simulink model "mechanical_system"  (R2015a)
settings: Solver=ode23t  StartTime=0.0  StopTime=10.0  RelTol=1e-3  AbsTol=1e-3
libraries: fl_lib x10, nesl_utility x4
settings Model: Creator=sseshadr  LastModifiedBy=sseshadr
settings SimscapeCC: SimscapeLogType=all  SimscapeLogDataHistory=10000

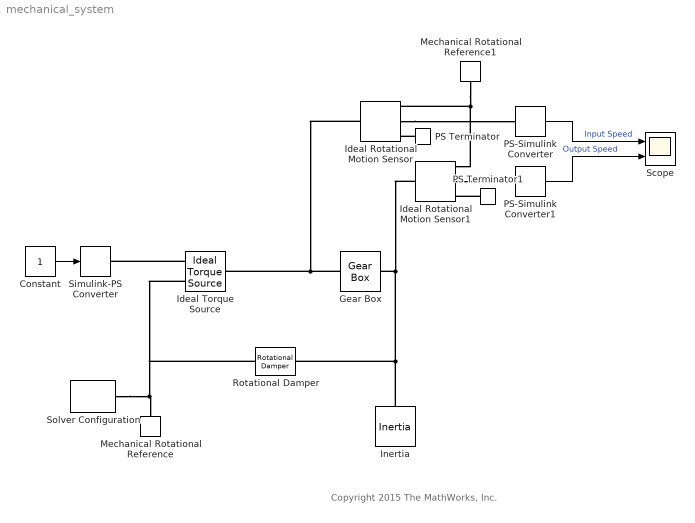
== system mechanical_system ==
  note: Copyright 2015 The MathWorks, Inc.
  Constant : Constant
  Gear Box : fl_lib/Mechanical/Mechanisms/Gear Box  ratio=2  t_in_specify=off  t_in_priority=High  t_in=0 N*m  t_out_specify=off  t_out_priority=High  t_out=0 N*m
  Ideal Rotational Motion Sensor : fl_lib/Mechanical/Mechanical Sensors/Ideal Rotational Motion Sensor  offset=0 rad
  Ideal Rotational Motion Sensor1 : fl_lib/Mechanical/Mechanical Sensors/Ideal Rotational Motion Sensor  offset=0 rad
  Ideal Torque Source : fl_lib/Mechanical/Mechanical Sources/Ideal Torque Source
  Inertia : fl_lib/Mechanical/Rotational Elements/Inertia  inertia=0.01 kg*m^2  w_specify=on  w_priority=High  w=10 rad/s  t_specify=off  t_priority=High  t=0 N*m
  Mechanical Rotational Reference : fl_lib/Mechanical/Rotational Elements/Mechanical Rotational Reference
  Mechanical Rotational Reference1 : fl_lib/Mechanical/Rotational Elements/Mechanical Rotational Reference
  PS Terminator : fl_lib/Physical Signals/Sinks/PS Terminator
  PS Terminator1 : fl_lib/Physical Signals/Sinks/PS Terminator
  PS-Simulink Converter : nesl_utility/PS-Simulink Converter  PhysicalDomain=network_engine_domain  SubClassName=ps_output  LeftPortType=input  RightPortType=output  PseudoPeriodic=off  Frequencies=[]  Unit=1  AffineConversion=off
  PS-Simulink Converter1 : nesl_utility/PS-Simulink Converter  PhysicalDomain=network_engine_domain  SubClassName=ps_output  LeftPortType=input  RightPortType=output  PseudoPeriodic=off  Frequencies=[]  Unit=1  AffineConversion=off
  Rotational Damper : fl_lib/Mechanical/Rotational Elements/Rotational Damper  D=0.001 N*m/(rad/s)  w_specify=off  w_priority=High  w=0 rad/s  t_specify=off  t_priority=High  t=0 N*m
  Scope : Scope  NumInputPorts=2
      settings: YMin=-5~-5  YMax=5~5
  Simulink-PS Converter : nesl_utility/Simulink-PS Converter  PhysicalDomain=network_engine_domain  SubClassName=ps_input  LeftPortType=input  RightPortType=output  PseudoPeriodic=off  Frequencies=[]  NoiseDistribution=none  NoiseParameters=[]  Unit=1  AffineConversion=off  InputFiltering=off  SimscapeFilterOrder=1  InputFilterTimeConstant=0.001  UdotUserProvided=1
  Solver Configuration : nesl_utility/Solver Configuration  PhysicalDomain=network_engine_domain  SubClassName=solver  LeftPortType=input  RightPortType=generic  Accelerate=off  Tones=[]  Harmonics=[]  SimulateNoise=off  Profile=off  UseLocalSampling=off  EnableSwitchedLinearOptims=on  FrequencyDomain=off  UseCCode=off  RelTol=0.001  AbsTol=1e-06  MinStep=1e-09  ToWorkspace=off  RevertToSquareIcSolve=off  NumHomotopyIterations=100  DoDC=off  ResidualTolerance=1e-09  UseLocalSolver=off  LocalSolverChoice=NE_BACKWARD_EULER_ADVANCER  LocalSolverSampleTime=0.001  DoFixedCost=off  MaxNonlinIter=3  MaxModeIter=2  LinearAlgebra=Sparse  DelaysMemoryBudget=1024  AutomaticFiltering=on  FilteringTimeConstant=0.001
  wires:
  PS-Simulink Converter/1 -> Scope/1  "Input Speed"
  Constant/1 -> Simulink-PS Converter/1
  PS-Simulink Converter1/1 -> Scope/2  "Output Speed"
  connections:
  Ideal Torque Source/RConn1 -- Simulink-PS Converter/RConn1
  Solver Configuration/RConn1 -- Ideal Torque Source/RConn2 -- Rotational Damper/RConn1 -- Mechanical Rotational Reference/LConn1
  Ideal Rotational Motion Sensor/LConn1 -- Ideal Torque Source/LConn1 -- Gear Box/LConn1
  Inertia/LConn1 -- Gear Box/RConn1 -- Ideal Rotational Motion Sensor1/LConn1 -- Rotational Damper/LConn1
  Ideal Rotational Motion Sensor/RConn2 -- PS-Simulink Converter/LConn1
  Ideal Rotational Motion Sensor1/RConn2 -- PS-Simulink Converter1/LConn1
  Mechanical Rotational Reference1/LConn1 -- Ideal Rotational Motion Sensor/RConn1 -- Ideal Rotational Motion Sensor1/RConn1
  PS Terminator/LConn1 -- Ideal Rotational Motion Sensor/RConn3
  PS Terminator1/LConn1 -- Ideal Rotational Motion Sensor1/RConn3
